simulink model "Q2"  (R2025a)
settings: Solver=ode45  StartTime=0.0  StopTime=10.0  MaxStep=0.001  RelTol=1e-3
settings Model: Creator=64892  LastModifiedBy=64892
settings DataIOCC: SaveFormat=StructureWithTime

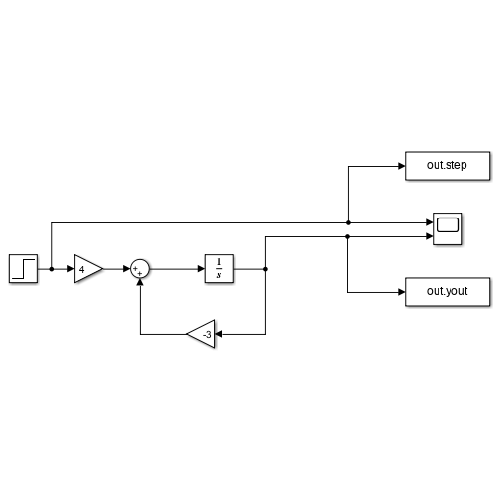
[thumbnail: Simulink's stored preview of the top-level diagram]
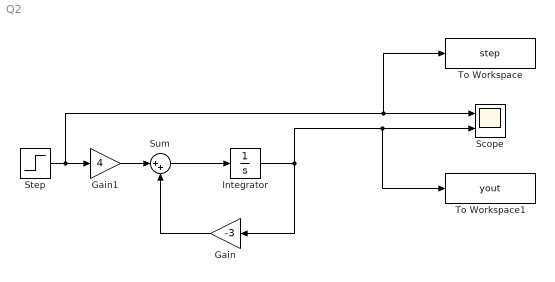
== system Q2 ==
  Gain : Gain  Gain=-3
  Gain1 : Gain  Gain=4
  Integrator : Integrator  InitialCondition=1
  Scope : Scope  NumInputPorts=2
      settings: ActiveDisplayYMinimum=-0.166666666666651  ActiveDisplayYMaximum=1.4999999999998592
  Step : Step  Time=0  SampleTime=0
  Sum : Sum  Inputs=|++
  To Workspace : ToWorkspace  VariableName=step  SaveFormat=Timeseries  SampleTime=-1
  To Workspace1 : ToWorkspace  VariableName=yout  SaveFormat=Timeseries  SampleTime=-1
  wires:
  Step/1 -> To Workspace/1, Scope/1, Gain1/1
  Gain1/1 -> Sum/1
  Sum/1 -> Integrator/1
  Integrator/1 -> To Workspace1/1, Scope/2, Gain/1
  Gain/1 -> Sum/2
